simulink model "HIB"  (R2021a)
settings: Solver=VariableStepAuto  StartTime=0.0  StopTime=10.0  RelTol=1e-3
settings Model: Creator=heyka  LastModifiedBy=heyka

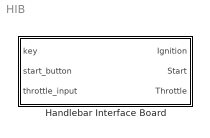
== system HIB ==
  Handlebar Interface Board : Stateflow chart  TreatAsAtomicUnit=on

== stateflow chart HIB/Handlebar Interface Board ==
  state Ignition_OFF
    during:
    Ignition = 0
    Throttle = 0
    Start = 0
  state Ignition_ON
    during:
    Ignition = 1
    Start = 0
  state Bike_Start
    during:
    Ignition = 1
    Start = 1
    Throttle = throttle_input
  (default) -> Ignition_OFF
  Ignition_OFF -> Ignition_ON : [key == 1]
  Ignition_ON -> Ignition_OFF [order 2] : [key == 0]
  Bike_Start -> Ignition_ON [order 1] : [start_button == 0]
  Ignition_ON -> Bike_Start [order 1] : [start_button== 1]
  Bike_Start -> Ignition_OFF [order 2] : [key == 0]
  data: Ignition output; Start output; key input; start_button input; Throttle output; throttle_input input
